simulink model "cruise_control_sdo_MILSIL"  (R2012b)
settings: Solver=FixedStepDiscrete  SolverMode=SingleTasking  StartTime=0  StopTime=0.14000000000000001  FixedStep=0.01  RelTol=1e-3  AbsTol=1e-6
model workspace (MAT data in the model file):
  converter_data = [0  137.465208994  2.232; 0.1  137.065019157  2.075; 0.2  135.864449646  1.975; 0.3  135.664354728  1.846; 0.4  137.565256453  1.72; 0.5  140.366585312  1.564; 0.6  145.268910814  1.409; 0.7  152.872517717  1.254; 0.8  162.9773111  1.096; 0.81  164.27792807  1.08; 0.82  166.178829795  1.061; 0.83  167.979684062  1.043; 0.84  170.080680706  1.028; 0.85  172.781962105  1.012; 0.86  175.383196045  1.002; 0.87  179.585189333  1.002; 0.88  183.587087703  1.001; 0.89  189.890077635  0.998; 0.9  197.693779455  0.999; 0.92  215.902417037  1.001; 0.94  244.515990379  1.002]
  emap = [-40  -44  -49  -53  -57  -61  -65  -70  -74  -78  -82; 215  117  85  66  44  29  10  -2  -13  -22  -32; 245  208  178  148  122  104  85  66  48  33  18; 264  260  241  219  193  167  152  133  119  96  85; 264  279  282  275  260  238  223  208  189  171  152; 267  290  293  297  290  275  260  256  234  212  193; 267  297  305  305  305  301  293  282  267  249  226; 267  301  308  312  319  323  319  316  297  279  253; 267  301  312  319  327  327  327  327  312  293  267; 267  301  312  319  327  334  334  334  319  305  275]
  Iei = 0.0219914882836
  nevec = [800 1200 1600 2000 2400 2800 3200 3600 4000 4400 4800]
  p0 = 0.07934
  p1 = 0.07934
  thvec = [0; 20; 30; 40; 50; 60; 70; 80; 90; 100]
  vehicledata = [3.23; 40; 0.3; 1; 50; 0]
undefined symbols (not defined in the file or in its folder): sigbuilder_block
undefined symbols (not defined in the file): throt_max, throt_min, vel_dec, vel_inc
libraries: simulink x3
settings Model: MinMaxOverflowLogging=MinMaxAndOverflow  SldvGeneratedHarnessModel=TestUnitModel=cruise_control_sdo|  CovMetricSettings=dcmoe  CovHTMLOptions=-aTS=1 -bRG=1 -bTC=0 -hTR=0 -nFC=0 -scm=1 -bcm=1  CovModelRefEnable=on  CovExternalEMLEnable=on  ExtModeTrigMode=oneshot  ExtModeArmWhenConnect=off  ExtModeAutoUpdateStatusClock=off  Creator=The MathWorks Inc.  LastModifiedBy=hualongy
settings DataIOCC: LimitDataPoints=off  SaveFormat=StructureWithTime  SignalLoggingSaveFormat=ModelDataLogs  SaveOutput=off  SaveTime=off  SignalLoggingName=mysig
settings OptimizationCC: BlockReduction=off  InlineParams=on  UseIntDivNetSlope=on  UseSpecifiedMinMax=on  InlineInvariantSignals=on  EnhancedBackFolding=on  ExpressionFolding=off  PassReuseOutputArgsAs=Individual arguments  ZeroExternalMemoryAtStartup=off  ZeroInternalMemoryAtStartup=off  NoFixptDivByZeroProtection=on  EfficientFloat2IntCast=on  OptimizeModelRefInitCode=on  LifeSpan=1
settings DebuggingCC: SignalInfNanChecking=error  SaveWithParameterizedLinksMsg=none  CheckExecutionContextPreStartOutputMsg=on  CheckExecutionContextRuntimeOutputMsg=on  SolverPrmCheckMsg=none  InheritedTsInSrcMsg=none  SingleTaskRateTransMsg=error  IntegerOverflowMsg=error  FcnCallInpInsideContextMsg=EnableAllAsWarning  UniqueDataStoreMsg=error  BusObjectLabelMismatch=error  RootOutportRequireBusObject=error  AssertControl=EnableAll  StrictBusMsg=ErrorOnBusTreatedAsVector  BusNameAdapt=ErrorWithoutRepair  NonBusSignalsTreatedAsBus=error  LoggingUnavailableSignals=none
settings HardwareCC: ProdIntDivRoundTo=Zero  ProdEndianess=LittleEndian  ProdHWDeviceType=NEC->V850  TargetIntDivRoundTo=Zero  TargetEndianess=LittleEndian  TargetHWDeviceType=MATLAB Host
settings ModelReferenceCC: ModelReferenceNumInstancesAllowed=Single
settings SFSimCC: SFSimEcho=off  SimParseCustomCode=off
settings RTWCC: SystemTargetFile=ert.tlc  GenCodeOnly=on  TemplateMakefile=ert_default_tmf  Description=Embedded Coder  GenerateReport=on  ProcessScript=ert_make_rtw_hook  IncludeHyperlinkInReport=on  LaunchReport=on  IncludeERTFirstTime=on  GenerateTraceInfo=on  GenerateTraceReport=on  GenerateTraceReportSl=on  GenerateTraceReportSf=on  GenerateTraceReportEml=on  RTWCompilerOptimization=On
settings CodeAppCC: IgnoreCustomStorageClasses=off  IgnoreTestpoints=on
settings ERTTargetCC: CodeReplacementLibrary=ANSI_C  UtilityFuncGeneration=Shared location  MultiwordLength=2048  GenerateSampleERTMain=on  IncludeMdlTerminateFcn=off  CombineSignalStateStructs=on  SuppressErrorStatus=on  SupportNonFinite=off  SupportComplex=off  PurelyIntegerCode=on  ParenthesesLevel=Maximum  InlinedParameterPlacement=NonHierarchical  ERTCustomFileTemplate=example_file_process.tlc  SuppressUnreachableDefaultCases=off
settings ConfigComp: Description=Design Verifier Custom Configuration Component  DVMaxProcessTime=3000  DVDisplayUnsatisfiableObjectives=on  DVMakeOutputFilesUnique=off  DVModelCoverageObjectives=MCDC  DVMaxTestCaseSteps=500  DVTestSuiteOptimization=CombinedObjectives (Nonlinear Extended)  DVSaveExpectedOutput=on  DVSaveHarnessModel=on  DVModelReferenceHarness=on  DVSaveReport=on

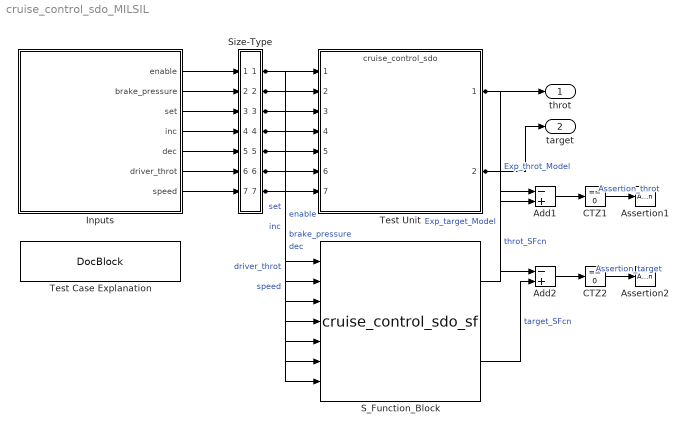
== system cruise_control_sdo_MILSIL ==
  Add1 : Sum  Inputs=-+  AccumDataTypeStr=double  OutDataTypeStr=double  SaturateOnIntegerOverflow=on  InputSameDT=on
  Add2 : Sum  Inputs=-+  AccumDataTypeStr=double  OutDataTypeStr=double  SaturateOnIntegerOverflow=on  InputSameDT=on
  Assertion1 : Assertion  Enabled=on  StopWhenAssertionFail=off
  Assertion2 : Assertion  Enabled=on  StopWhenAssertionFail=off
  CTZ1 : simulink/Logic and Bit Operations/Compare To Zero  relop===  OutDataTypeStr=boolean
  CTZ2 : simulink/Logic and Bit Operations/Compare To Zero  relop===  OutDataTypeStr=boolean
  Inputs : Subsystem  Tag=STV Subsys  LoadFcn=sigbuilder_block('load',[49.5 50.25 519.75 399.75 ]);  StartFcn=sigbuilder_block('start');  StopFcn=sigbuilder_block('stop');  ClipboardFcn=sigbuilder_block('clipboard');  mask(Sigbuilder block){}
      mask init:
      | if ~strcmp(get_param(bdroot(gcb),'SimulationStatus'),'stopped'),tuvar = sigbuilder_block('maskInit'); end
      settings: CopyFcn=sigbuilder_block('copy');  DeleteFcn=sigbuilder_block('delete');  ModelCloseFcn=sigbuilder_block('modelClose');  PreSaveFcn=sigbuilder_block('preSave');  PauseFcn=sigbuilder_block('pause');  ContinueFcn=sigbuilder_block('continue');  NameChangeFcn=sigbuilder_block('namechange');  OpenFcn=sigbuilder_block('open');  CloseFcn=sigbuilder_block('close');
      mask Display: plot(0, 0, 100, 100,[2, 2, 32, 32, 2], [68, 8, 8, 68, 68],[32, 2], [38, 38], [32, 19, 2],[53, 60, 44], [32, 17, 17, 2],[16, 16, 31, 31]);txt = getActiveGroup(gcbh);text(2, 100, txt,'verticalAlignment', 'top');
  S_Function_Block : S-Function  FunctionName=cruise_control_sdo_sf  Parameters=sfcnParam1, sfcnParam2, sfcnParam3, sfcnParam4  SFunctionModules=""  EnableBusSupport=off  mask{rtw_sf_name=cruise_control_sdo_sf, showVar=off, sfcnParam1=throt_max, sfcnParam2=throt_min, sfcnParam3=vel_dec, sfcnParam4=vel_inc}
      mask prompts: rtw_sf_name "Simulink:masks:GenSFuncName_MP"; showVar "Simulink:masks:GenSFuncShowModuleList_MP"; sfcnParam1 "throt_max:"; sfcnParam2 "throt_min:"; sfcnParam3 "vel_dec:"; sfcnParam4 "vel_inc:"
      mask help: Simulink:masks:GenSFuncDesc_MD
      mask init:
      | displist = '';
      | if ~strcmp(get_param(gcb, 'FunctionName'), rtw_sf_name);
      |   set_param(gcb, 'FunctionName', rtw_sf_name);
      | end
      | % Check if we are generating code
      | rtw_mode = false;
      | if strcmpi(get_param(bdroot(gcb),'SimulationStatus'),'Initializing')
      | 	rtw_mode = strcmpi(get_param(bdroot(gcb),'BuildingRTWCode'),'on') && ...
      | 		~strcmpi(get_param(bdroot(gcb),'TargetStyle'),'SimulationTarget');
      | end
      | if showVar || rtw_mode
      | 	if exist('rtwsfunc') == 2 | exist('rtwsfunc') == 6
      | 		tmplist = rtwsfunc(rtw_sf_name,gcb);
      | 		tmplist = DAStudio.message('Simulink:masks:GenSFuncListOfModules_IC', tmplist);
      | 	elseif showVar
      | 		tmplist1 = DAStudio.message('Simulink:masks:GenSFuncListOfModules_IC', '');
      |         tmplist2 = DAStudio.message('Simulink:masks:GenSFuncNotLicensed_IC');
      |         tmplist = [tmplist1 tmplist2];
      |  	end
      | end
      | if showVar
      |   displist = tmplist;
      | end
      settings: CopyFcn=|
      | if ~strcmp(get_param(gcb,'Linkstatus'),'none') && ...
      | ~strcmp(get_param(gcb,'Linkstatus'),'implicit')
      |   set_param(gcb,'LinkStatus','none');
      | end
      mask Help: helpview([docroot '/toolbox/ecoder/helptargets.map'], 'SIL_block');
      mask Display:
      | port_label('input',1,'enable');
      | port_label('input',2,'brake_pressure');
      | port_label('input',3,'set');
      | port_label('input',4,'inc');
      | port_label('input',5,'dec');
      | port_label('input',6,'driver_throt');
      | port_label('input',7,'speed');
      | port_label('output',1,'throt');
      | port_label('output',2,'target');
  Size-Type : Subsystem
  Test Case Explanation : simulink/Model-Wide Utilities/DocBlock  DocumentType=Text
  Test Unit : ModelReference  ModelNameDialog=cruise_control_sdo  SimulationMode=Normal  ModelReferenceVersion=1.305  CopyOfModelName=cruise_control_sdo  DefaultDataLogging=off
  throt : Outport  PortDimensions=[1 1]
  target : Outport  Port=2  PortDimensions=[1 1]
  wires:
  Inputs/1(enable) -> Size-Type/1(In1)
  Size-Type/1(Out1) -> Test Unit/1, S_Function_Block/1  "enable"
  Inputs/2(brake_pressure) -> Size-Type/2(In2)
  Size-Type/2(Out2) -> Test Unit/2, S_Function_Block/2  "brake_pressure"
  Inputs/3(set) -> Size-Type/3(In3)
  Size-Type/3(Out3) -> Test Unit/3, S_Function_Block/3  "set"
  Inputs/4(inc) -> Size-Type/4(In4)
  Size-Type/4(Out4) -> Test Unit/4, S_Function_Block/4  "inc"
  Inputs/5(dec) -> Size-Type/5(In5)
  Size-Type/5(Out5) -> Test Unit/5, S_Function_Block/5  "dec"
  Inputs/6(driver_throt) -> Size-Type/6(In6)
  Size-Type/6(Out6) -> Test Unit/6, S_Function_Block/6  "driver_throt"
  Inputs/7(speed) -> Size-Type/7(In7)
  Size-Type/7(Out7) -> Test Unit/7, S_Function_Block/7  "speed"
  Test Unit/1 -> throt/1, Add1/1  "Exp_throt_Model"
  Test Unit/2 -> target/1, Add2/1  "Exp_target_Model"
  S_Function_Block/1 -> Add1/2  "throt_SFcn"
  Add1/1 -> CTZ1/1
  CTZ1/1 -> Assertion1/1  "Assertion_throt"
  S_Function_Block/2 -> Add2/2  "target_SFcn"
  Add2/1 -> CTZ2/1
  CTZ2/1 -> Assertion2/1  "Assertion_target"

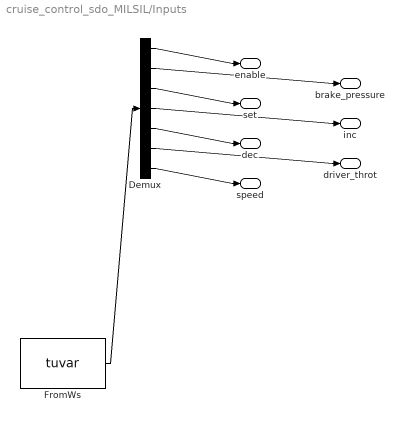
== system cruise_control_sdo_MILSIL/Inputs ==
  Demux : Demux  Tag=STV Demux  Outputs=7
  FromWs : FromWorkspace  Tag=STV FromWs  VariableName=tuvar  SampleTime=0
      SigBuilderData=|
      | dataSet.timeRange = [0 0.14]
      | dataSet.name = 'Test Case 1'
      | sbobj.Name = 'Signal Builder'
      | sbobj.Groups.Name = 'Test Case 1'
      | sbobj.Groups.Signals(1).Name = 'enable'
      | sbobj.Groups.Signals(1).XData = [0 0.01 0.02 0.03 0.04 0.05 0.05 0.06 0.07 0.08 0.09 0.09 0.1 0.11 0.12 0.12 0.13 0.14]
      | sbobj.Groups.Signals(1).YData = [0 0 0 0 0 0 1 1 1 1 1 0 0 0 0 1 1 1]
      | sbobj.Groups.Signals(2).Name = 'brake_pressure'
      | sbobj.Groups.Signals(2).XData = [0 0.01 0.01 0.02 0.02 0.03 0.03 0.04 0.04 0.05 0.05 0.06 0.06 0.07 0.07 0.08 0.08 0.09 0.09 0.1 0.1 0.11 0.11 0.12 0.12 0.13 0.13 0.14]
      | sbobj.Groups.Signals(2).YData = [2.875 2.875 0 0 0 0 0 0 0 0 0 0 0.0625 0.0625 0 0 0 0 0 0 0 0 0 0 8 8 0 0]
      | sbobj.Groups.Signals(3).Name = 'set'
      | sbobj.Groups.Signals(3).XData = [0 0.01 0.01 0.02 0.02 0.03 0.03 0.04 0.04 0.05 0.05 0.06 0.06 0.07 0.07 0.08 0.08 0.09 0.09 0.1 0.1 0.11 0.11 0.12 0.12 0.13 0.13 0.14]
      | sbobj.Groups.Signals(3).YData = [1 1 0 0 0 0 0 0 0 0 0 0 0 0 1 1 1 1 0 0 0 0 1 1 1 1 0 0]
      | sbobj.Groups.Signals(4).Name = 'inc'
      | sbobj.Groups.Signals(4).XData = [0 0.01 0.01 0.02 0.02 0.03 0.03 0.04 0.04 0.05 0.05 0.06 0.06 0.07 0.07 0.08 0.08 0.09 0.09 0.1 0.1 0.11 0.11 0.12 0.12 0.13 0.13 0.14]
      | sbobj.Groups.Signals(4).YData = [1 1 0 0 1 1 0 0 0 0 0 0 0 0 0 0 0 0 0 0 0 0 0 0 0 0 0 0]
      | sbobj.Groups.Signals(5).Name = 'dec'
      | sbobj.Groups.Signals(5).XData = [0 0.01 0.01 0.02 0.02 0.03 0.03 0.04 0.04 0.05 0.05 0.06 0.06 0.07 0.07 0.08 0.08 0.09 0.09 0.1 0.1 0.11 0.11 0.12 0.12 0.13 0.13 0.14]
      | sbobj.Groups.Signals(5).YData = [0 0 0 0 0 0 0 0 1 1 0 0 0 0 0 0 0 0 0 0 0 0 0 0 0 0 0 0]
      | sbobj.Groups.Signals(6).Name = 'driver_throt'
      | sbobj.Groups.Signals(6).XData = [0 0.01 0.01 0.02 0.02 0.03 0.03 0.04 0.04 0.05 0.05 0.06 0.06 0.07 0.07 0.08 0.08 0.09 0.09 0.1 0.1 0.11 0.11 0.12 0.12 0.13 0.13 0.14]
      | sbobj.Groups.Signals(6).YData = [4.9375 4.9375 0 0 0 0 0 0 0 0 0 0 0 0 0 0 0 0 0 0 100 100 0 0 0 0 0 0]
      | sbobj.Groups.Signals(7).Name = 'speed'
      | sbobj.Groups.Signals(7).XData = [0 0.01 0.01 0.02 0.02 0.03 0.03 0.04 0.04 0.05 0.05 0.06 0.06 0.07 0.07 0.08 0.08 0.09 0.09 0.1 0.1 0.11 0.11 0.12 0.12 0.13 0.13 0.14]
      | sbobj.Groups.Signals(7).YData = [6.125 6.125 256 256 256 256 46 46 256 256 256 256 256 256 256 256 46 46 256 256 256 256 46 46 46 46 46 46]
      | sbobj.Groups.TimeRange = [0 0.14]
  enable : Outport  Tag=STV Outport
  brake_pressure : Outport  Tag=STV Outport  Port=2
  set : Outport  Tag=STV Outport  Port=3
  inc : Outport  Tag=STV Outport  Port=4
  dec : Outport  Tag=STV Outport  Port=5
  driver_throt : Outport  Tag=STV Outport  Port=6
  speed : Outport  Tag=STV Outport  Port=7
  wires:
  FromWs/1 -> Demux/1
  Demux/1 -> enable/1
  Demux/2 -> brake_pressure/1
  Demux/3 -> set/1
  Demux/4 -> inc/1
  Demux/5 -> dec/1
  Demux/6 -> driver_throt/1
  Demux/7 -> speed/1

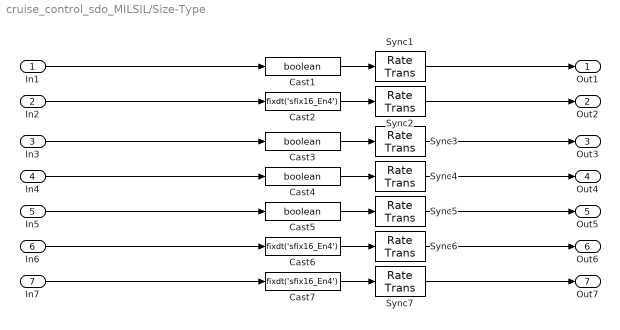
== system cruise_control_sdo_MILSIL/Size-Type ==
  In1 : Inport
  In2 : Inport  Port=2
  In3 : Inport  Port=3
  In4 : Inport  Port=4
  In5 : Inport  Port=5
  In6 : Inport  Port=6
  In7 : Inport  Port=7
  Cast{1,3..5} (4 alike) : DataTypeConversion  OutDataTypeStr=boolean  SaturateOnIntegerOverflow=on  RndMeth=Zero
  Cast2 : DataTypeConversion  OutDataTypeStr=fixdt('sfix16_En4')  SaturateOnIntegerOverflow=on  RndMeth=Zero
  Cast6 : DataTypeConversion  OutDataTypeStr=fixdt('sfix16_En4')  SaturateOnIntegerOverflow=on  RndMeth=Zero
  Cast7 : DataTypeConversion  OutDataTypeStr=fixdt('sfix16_En4')  SaturateOnIntegerOverflow=on  RndMeth=Zero
  Sync{1..7} (7 alike) : RateTransition  OutPortSampleTime=[0.01,0]
  Out1 : Outport
  Out2 : Outport  Port=2
  Out3 : Outport  Port=3
  Out4 : Outport  Port=4
  Out5 : Outport  Port=5
  Out6 : Outport  Port=6
  Out7 : Outport  Port=7
  wires:
  In1/1 -> Cast1/1
  Cast1/1 -> Sync1/1
  Sync1/1 -> Out1/1
  In2/1 -> Cast2/1
  Cast2/1 -> Sync2/1
  Sync2/1 -> Out2/1
  In3/1 -> Cast3/1
  Cast3/1 -> Sync3/1
  Sync3/1 -> Out3/1
  In4/1 -> Cast4/1
  Cast4/1 -> Sync4/1
  Sync4/1 -> Out4/1
  In5/1 -> Cast5/1
  Cast5/1 -> Sync5/1
  Sync5/1 -> Out5/1
  In6/1 -> Cast6/1
  Cast6/1 -> Sync6/1
  Sync6/1 -> Out6/1
  In7/1 -> Cast7/1
  Cast7/1 -> Sync7/1
  Sync7/1 -> Out7/1
